simulink model "twiddle_pass_through_test"  (Simulink 7.4)
settings: Solver=VariableStepDiscrete  StartTime=0.0  StopTime=1000  RelTol=1e-3
libraries: xbsIndex_r4 x9, casper_library_misc x1
settings Model: Creator=User  LastModifiedBy=mwagner
settings OptimizationCC: InitFltsAndDblsToZero=on
settings DebuggingCC: SaveWithDisabledLinksMsg=none  SaveWithParameterizedLinksMsg=none

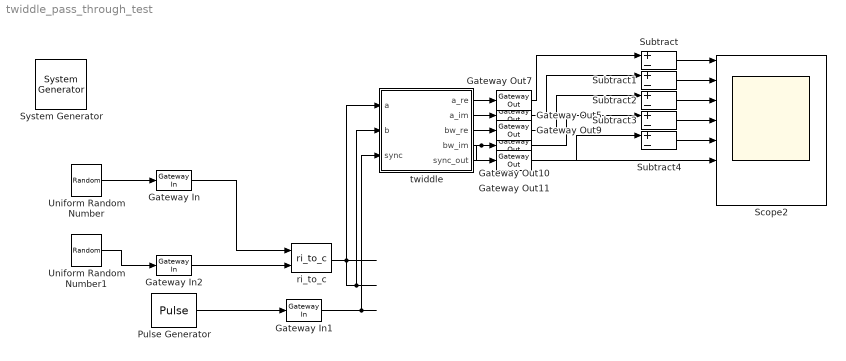
== system twiddle_pass_through_test ==
  " System Generator" : xbsIndex_r4/ System Generator  Tag=genX  SystemSampleTime=-1  xilinxfamily=Virtex4  part=xc4vsx35  speed=-10  package=ff668  synthesis_tool=XST  clock_wrapper=Clock Enables  directory=./netlist  testbench=off  simulink_period=1  sysclk_period=100  dcm_input_clock_period=100  incr_netlist=off  trim_vbits=Everywhere in SubSystem  dbl_ovrd=According to Block Masks  core_generation=According to Block Masks  run_coregen=off  deprecated_control=off  eval_field=0  block_type=sysgen
      settings: block_version=10.1.1
  Gateway In : xbsIndex_r4/Gateway In  arith_type="Signed  (2's comp)"  n_bits=5  bin_pt=4  quantization=Truncate  overflow=Wrap  period=1  dbl_ovrd=off  timing_constraint=None  locs_specified=off  LOCs={}  hdl_port=on  block_type=gatewayin
      settings: infoedit="Gateway in block.  Converts inputs of type Simulink integer, double and fixed point to  Xilinx fixed point type.<P><P>Hardware notes:  In hardware these blocks become top level input ports."  block_version=10.1.1
  Gateway In1 : xbsIndex_r4/Gateway In  arith_type=Boolean  n_bits=16  bin_pt=14  quantization="Round  (unbiased: +/- Inf)"  overflow=Saturate  period=1  dbl_ovrd=off  timing_constraint=None  locs_specified=off  LOCs={}  hdl_port=on  block_type=gatewayin
      settings: infoedit="Gateway in block.  Converts inputs of type Simulink integer, double and fixed point to  Xilinx fixed point type.<P><P>Hardware notes:  In hardware these blocks become top level input ports."  block_version=10.1.1
  Gateway In2 : xbsIndex_r4/Gateway In  arith_type="Signed  (2's comp)"  n_bits=5  bin_pt=4  quantization=Truncate  overflow=Wrap  period=1  dbl_ovrd=off  timing_constraint=None  locs_specified=off  LOCs={}  hdl_port=on  block_type=gatewayin
      settings: infoedit="Gateway in block.  Converts inputs of type Simulink integer, double and fixed point to  Xilinx fixed point type.<P><P>Hardware notes:  In hardware these blocks become top level input ports."  block_version=10.1.1
  Gateway Out{5,7,9..11} (5 alike) : xbsIndex_r4/Gateway Out  hdl_port=on  timing_constraint=None  locs_specified=off  LOCs={}  block_type=gatewayout
      settings: infoedit="Gateway out block.  Converts Xilinx fixed point inputs into ouputs of type Simulink integer, double, or fixed point.<P><P>Hardware notes:  In hardware these blocks become top level output ports or are discarded, depending on how they are configured."  block_version=10.1.1
  Pulse Generator : DiscretePulseGenerator  Amplitude=1  Period=256  PulseWidth=1  PhaseDelay=7  SampleTime=1
  Scope2 : Scope  NumInputPorts=8
      settings: TimeRange=1000  YMin=-1~0~-1~-1~0~-1~-1~-1  YMax=1~1~1~1~1~1~1~1  SaveName=ScopeData2
  Subtract{,1..4} (5 alike) : Sum  Inputs=+-  OutDataType=fixdt(1, 16)  OutScaling=2^-10
  Uniform Random Number : UniformRandomNumber  SampleTime=1
  Uniform Random Number1 : UniformRandomNumber  Seed=1  SampleTime=1
  ri_to_c : casper_library_misc/ri_to_c  SystemSampleTime=-1
  twiddle : Subsystem  mask(fft_twiddle){FFTSize=6, Coeffs=[0], StepPeriod=4, input_bit_width=5, coeff_bit_width=18, add_latency=2, mult_latency=3, bram_latency=2, conv_latency=1, input_latency=0, mux_latency=8, negate_latency=3, arch=Virtex5, coeffs_bram=on, use_hdl=off, use_embedded=off, quantization=Truncate, overflow=Wrap, opt_target='Logic', use_dsp48_mults=0, biplex=on}
      mask prompts: FFTSize "FFT Size"; Coeffs "Coefficients:"; StepPeriod "Coefficient Step Period (2^?)"; input_bit_width "Input Bit Width"; coeff_bit_width "Coefficient Bit Width"; add_latency "Add Latency"; mult_latency "Multiply Latency"; bram_latency "BRAM Latency"; conv_latency "Convert Latency"; input_latency "Input Latency"; arch "Architecture"; coeffs_bram "Store coefficients in BRAM"; use_hdl "Use HDL Arithmetic"; use_embedded "Use Embedded Arithmetic"; quantization "Quantization Behavior"; overflow "Overflow Behavior"; opt_target "Optimization Target"; use_dsp48_mults "Use DSP48E multipliers"; biplex "Biplex?"
      mask help:
      | Used in biplex pipelined FFT.
      |
      | Computes (ac-bd)+i(ad+bc) using 4 DSP48Es.
      mask init:
      | config.source = str2func('fft_twiddle_init_xblock');
      | config.toplevel = gcb;
      | 
      | xBlock(config, {...
      |     'FFTSize', FFTSize, ...
      |     'Coeffs', Coeffs, ...
      |     'StepPeriod', StepPeriod, ...
      |     'input_bit_width', input_bit_width, ...    
      |     'coeff_bit_width', coeff_bit_width, ...
      |     'add_latency', add_latency, ...
      |     'mult_latency', mult_latency, ...
      |     'bram_latency', bram_latency, ...
      |     'conv_latency', conv_latency, ...
      |     'input_latency', input_latency, ...
      |     'mux_latency', mux_latency, ...
      |     'negate_latency', negate_latency, ...
      |     'arch', arch, ...
      |     'coeffs_bram', coeffs_bram ...
      |     'use_hdl', use_hdl, ...
      |     'use_embedded', use_embedded, ...
      |     'quantization', quantization, ...
      |     'overflow', overflow, ...
      |     'opt_target', opt_target, ...
      |     'use_dsp48_mults', use_dsp48_mults, ... 
      |     'biplex', biplex, ...
      |     } );
      settings: AttributesFormatString=|
      | data=(18,17)
      | coeffs=(18,16)
      | Virtex5
      | (Round  (unbiased: +/- Inf),Wrap)
      mask StyleString: edit,edit,edit,edit,edit,edit,edit,edit,edit,edit,edit,edit,popup(Virtex5),checkbox,checkbox,checkbox,popup(Truncate|Round  (unbiased: +/- Inf)|Round  (unbiased: Even Values)),popup(Wrap|Saturate|Error),edit,edit,checkbox
      mask TabNameString: Basic,Basic,Basic,Basic,Basic,Latency,Latency,Latency,Latency,Latency,Latency,Latency,Implementation,Implementation,Implementation,Implementation,Implementation,Implementation,Implementation,Implementation,Implementation
  wires:
  Uniform Random Number/1 -> Gateway In/1
  Pulse Generator/1 -> Gateway In1/1
  Gateway In1/1 -> twiddle/3(sync)
  Gateway In/1 -> ri_to_c/1
  ri_to_c/1 -> twiddle/2(b), twiddle/1(a)
  Subtract/1 -> Scope2/1
  Subtract1/1 -> Scope2/2
  Subtract2/1 -> Scope2/3
  Subtract3/1 -> Scope2/4
  Subtract4/1 -> Scope2/5
  Gateway Out7/1 -> Subtract/1
  Gateway Out5/1 -> Subtract1/1
  Gateway Out9/1 -> Subtract2/1
  Gateway Out10/1 -> Subtract3/1
  Gateway Out11/1 -> Subtract4/1
  Uniform Random Number1/1 -> Gateway In2/1
  Gateway In2/1 -> ri_to_c/2
  twiddle/1(a_re) -> Gateway Out7/1
  twiddle/2(a_im) -> Gateway Out5/1
  twiddle/3(bw_re) -> Gateway Out9/1
  twiddle/4(bw_im) -> Gateway Out10/1, Scope2/6
  twiddle/5(sync_out) -> Gateway Out11/1

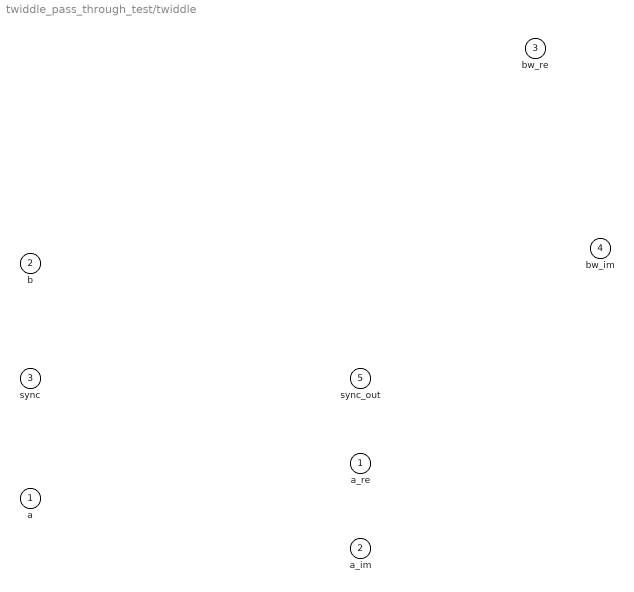
== system twiddle_pass_through_test/twiddle ==
  a : Inport
  b : Inport  Port=2
  sync : Inport  Port=3
  a_re : Outport
  a_im : Outport  Port=2
  bw_re : Outport  Port=3
  bw_im : Outport  Port=4
  sync_out : Outport  Port=5
